simulink model "model_8264"  (R2022b)
settings: Solver=FixedStepAuto  StartTime=0.0  StopTime=2.4  FixedStep=2e-5  RelTol=1e-3
undefined symbols (not defined in the file): Acid, Lead, sigbuilder_block
libraries: spsMeanLib x24, spsVoltageMeasurementLib x18, spsGroundLib x15, spsCurrentMeasurementLib x15, spsIdealSwitchLib x12, spsSeriesRLCLoadLib x12, spsSeriesRLCBranchLib x5, spsThreePhaseVIMeasurementLib x4, simulink x4, spsPower3phInstantaneousLib x3, spsThreePhaseBreakerLib x2, slpidlib x2
(part 2 of 2)

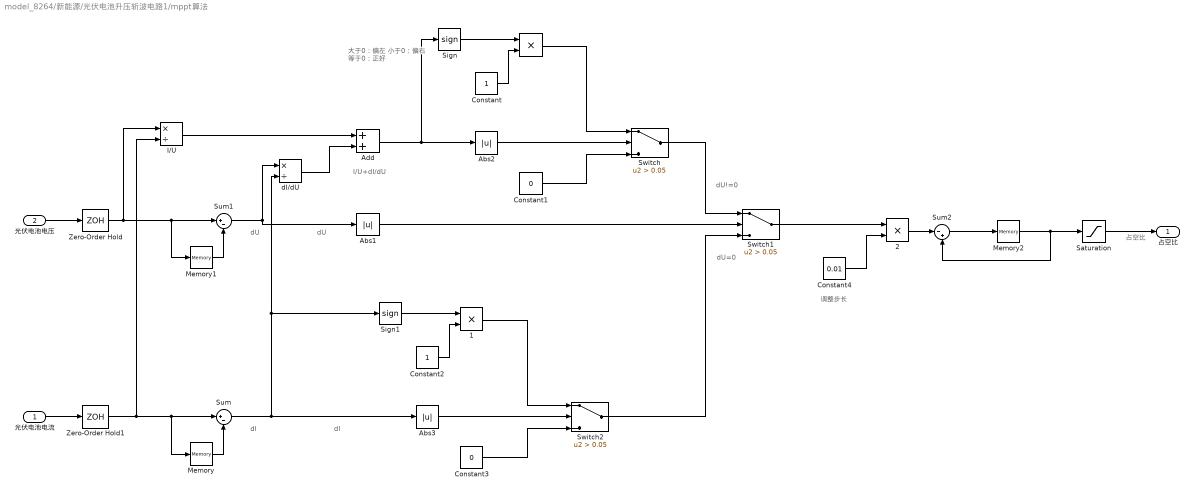
== system model_8264/新能源/光伏电池升压斩波电路1/mppt算法 ==
  note: dU!=0
  note: 占空比
  note: 调整步长
  note: 大于0：偏左
      | 小于0：偏右
      | 等于0：正好
  note: I/U+dI/dU
  note: dI
  note: dU
  note: dU
  note: dI
  note: dU=0
  光伏电池电流 : Inport
  光伏电池电压 : Inport  Port=2
  " " : Product  Inputs=**
  " 1" : Product  Inputs=**
  " 2" : Product  Inputs=**
  Abs1 : Abs  SaturateOnIntegerOverflow=off
  Abs2 : Abs  SaturateOnIntegerOverflow=off
  Abs3 : Abs  SaturateOnIntegerOverflow=off
  Add : Sum
  Constant : Constant
  Constant1 : Constant  Value=0
  Constant2 : Constant
  Constant3 : Constant  Value=0
  Constant4 : Constant  Value=0.01
  I/U : Product  Inputs=*/
  Memory : Memory
  Memory1 : Memory
  Memory2 : Memory  InitialCondition=0.5  InheritSampleTime=on
  Saturation : Saturate  UpperLimit=1  LowerLimit=0
  Sign : Signum
  Sign1 : Signum
  Sum : Sum  Inputs=|+-
  Sum1 : Sum  Inputs=|+-
  Sum2 : Sum  Inputs=|-+
  Switch : Switch  Criteria=u2 > Threshold  Threshold=0.05  SaturateOnIntegerOverflow=off  InputSameDT=off
  Switch1 : Switch  Criteria=u2 > Threshold  Threshold=0.05  SaturateOnIntegerOverflow=off  InputSameDT=off
  Switch2 : Switch  Criteria=u2 > Threshold  Threshold=0.05  SaturateOnIntegerOverflow=off  InputSameDT=off
  Zero-Order Hold : ZeroOrderHold  SampleTime=0.05
  Zero-Order Hold1 : ZeroOrderHold  SampleTime=0.05
  dI/dU : Product  Inputs=*/
  占空比 : Outport
  wires:
  光伏电池电流/1 -> Zero-Order Hold1/1
  光伏电池电压/1 -> Zero-Order Hold/1
  Zero-Order Hold1/1 -> I/U/2, Memory/1, Sum/1
  Memory/1 -> Sum/2
  Memory1/1 -> Sum1/2
  Sum1/1 -> dI/dU/1, Abs1/1
  Zero-Order Hold/1 -> I/U/1, Memory1/1, Sum1/1
  I/U/1 -> Add/1
  dI/dU/1 -> Add/2
  Add/1 -> Sign/1, Abs2/1
  Sign/1 -> " "/1
  Constant/1 -> " "/2
  Abs2/1 -> Switch/2
  Constant1/1 -> Switch/3
  " "/1 -> Switch/1
  Abs1/1 -> Switch1/2
  Switch/1 -> Switch1/1
  Sum/1 -> Abs3/1, Sign1/1, dI/dU/2
  Constant3/1 -> Switch2/3
  Constant2/1 -> " 1"/2
  Abs3/1 -> Switch2/2
  " 1"/1 -> Switch2/1
  Sign1/1 -> " 1"/1
  Switch2/1 -> Switch1/3
  Switch1/1 -> " 2"/1
  Constant4/1 -> " 2"/2
  " 2"/1 -> Sum2/1
  Sum2/1 -> Memory2/1
  Memory2/1 -> Sum2/2, Saturation/1
  Saturation/1 -> 占空比/1

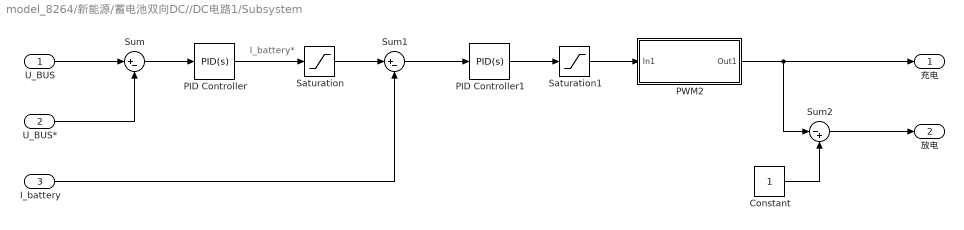
== system model_8264/新能源/蓄电池双向DC//DC电路1/Subsystem ==
  note: I_battery*
  U_BUS : Inport
  U_BUS* : Inport  Port=2
  I_battery : Inport  Port=3
  Constant : Constant
  PID Controller : slpidlib/PID Controller  Controller=PID  Form=Parallel  TimeDomain=Continuous-time  UseExternalTs=off  SampleTime=-1  IntegratorMethod=Forward Euler  FilterMethod=Forward Euler  ControllerParametersSource=internal  P=0.1  I=1  UseKiTs=off  D=0  N=100  UseFilter=on  TunerSelectOption=Transfer Function Based (PID Tuner App)  InitialConditionSource=internal  InitialConditionForIntegrator=0  InitialConditionForFilter=0  DifferentiatorICPrevScaledInput=0  ExternalReset=none  TrackingMode=off  Kt=1  LimitOutput=off  SatLimitsSource=internal  UpperSaturationLimit=inf  LowerSaturationLimit=-inf  LinearizeAsGain=on  AntiWindupMode=none  Kb=1  LimitIntegrator=off  UpperIntegratorSaturationLimit=inf  LowerIntegratorSaturationLimit=-inf  POutMin=[]  POutMax=[]  IOutMin=[]  IOutMax=[]  DOutMin=[]  DOutMax=[]  NOutMin=[]  NOutMax=[]  SumOutMin=[]  SumOutMax=[]  SaturationOutMin=[]  SaturationOutMax=[]  PParamMin=[]  PParamMax=[]  IParamMin=[]  IParamMax=[]  DParamMin=[]  DParamMax=[]  NParamMin=[]  NParamMax=[]  KbParamMin=[]  KbParamMax=[]  KtParamMin=[]  KtParamMax=[]  KbOutMin=[]  KbOutMax=[]  KtOutMin=[]  KtOutMax=[]  IntegratorOutMin=[]  IntegratorOutMax=[]  FilterOutMin=[]  FilterOutMax=[]  SumI1OutMin=[]  SumI1OutMax=[]  SumI2OutMin=[]  SumI2OutMax=[]  SumI3OutMin=[]  SumI3OutMax=[]  SumI4OutMin=[]  SumI4OutMax=[]  SumDOutMin=[]  SumDOutMax=[]  DifferentiatorOutMin=[]  DifferentiatorOutMax=[]  FilterDiffOutCoefMin=[]  FilterDiffOutCoefMax=[]  ReciprocalOutMin=[]  ReciprocalOutMax=[]  SumDenOutMin=[]  SumDenOutMax=[]  SumNumOutMin=[]  SumNumOutMax=[]  DivideOutMin=[]  DivideOutMax=[]  UdiffTsProdOutMin=[]  UdiffTsProdOutMax=[]  NTsProdOutMin=[]  NTsProdOutMax=[]  UintegralTsProdOutMin=[]  UintegralTsProdOutMax=[]  UngainTsProdOutMin=[]  UngainTsProdOutMax=[]  ClampingZeroOutDataTypeStr=Inherit: Inherit via back propagation  ClampingZeroOutMin=[]  ClampingZeroOutMax=[]  FilterDenConstantOutDataTypeStr=Inherit: Inherit via back propagation  FilterDenConstantOutMin=[]  FilterDenConstantOutMax=[]  PCopyOutDataTypeStr=Inherit: Inherit via back propagation  PCopyOutMin=[]  PCopyOutMax=[]  NCopyOutDataTypeStr=Inherit: Inherit via back propagation  NCopyOutMin=[]  NCopyOutMax=[]  IntegratorContinuousStateAttributes=''  IntegratorStateMustResolveToSignalObject=off  IntegratorRTWStateStorageClass=Auto  FilterContinuousStateAttributes=''  FilterStateMustResolveToSignalObject=off  FilterRTWStateStorageClass=Auto  ParallelPVariant=InternalParameters  IdealPVariant=Disabled  IVariant=InternalParameters  DVariant=InternalParameters  IntegratorVariant=Continuous  SatVariant=Disabled  AWVariant=Passthrough  PCopyVariant=Disabled  TRVariant=Disabled  FdbkBlocksVariant=Forward  IdealPFdbkVariant=Disabled  SatFdbkVariant=Disabled  DerivativeFilterVariant=ContFilter  NVariant=InternalParameters  NCopyVariant=Disabled  FilterICVariant=InternalICsFilter  IntegratorICVariant=InternalICs  ExternalResetVariant=Disabled  TRSumVariant=Passthrough  SumFdbkVariant=Disabled  SumVariant=Sum_PID  TsampFilterVariant=InternalTs  TsampNgainVariant=Passthrough  TsampIntegralVariant=Passthrough  ExternalSaturationOutDataTypeStr=Inherit: Same as second input
  PID Controller1 : slpidlib/PID Controller  Controller=PID  Form=Parallel  TimeDomain=Continuous-time  UseExternalTs=off  SampleTime=-1  IntegratorMethod=Forward Euler  FilterMethod=Forward Euler  ControllerParametersSource=internal  P=0.02  I=1  UseKiTs=off  D=0  N=100  UseFilter=on  TunerSelectOption=Transfer Function Based (PID Tuner App)  InitialConditionSource=internal  InitialConditionForIntegrator=0  InitialConditionForFilter=0  DifferentiatorICPrevScaledInput=0  ExternalReset=none  TrackingMode=off  Kt=1  LimitOutput=off  SatLimitsSource=internal  UpperSaturationLimit=inf  LowerSaturationLimit=-inf  LinearizeAsGain=on  AntiWindupMode=none  Kb=1  LimitIntegrator=off  UpperIntegratorSaturationLimit=inf  LowerIntegratorSaturationLimit=-inf  POutMin=[]  POutMax=[]  IOutMin=[]  IOutMax=[]  DOutMin=[]  DOutMax=[]  NOutMin=[]  NOutMax=[]  SumOutMin=[]  SumOutMax=[]  SaturationOutMin=[]  SaturationOutMax=[]  PParamMin=[]  PParamMax=[]  IParamMin=[]  IParamMax=[]  DParamMin=[]  DParamMax=[]  NParamMin=[]  NParamMax=[]  KbParamMin=[]  KbParamMax=[]  KtParamMin=[]  KtParamMax=[]  KbOutMin=[]  KbOutMax=[]  KtOutMin=[]  KtOutMax=[]  IntegratorOutMin=[]  IntegratorOutMax=[]  FilterOutMin=[]  FilterOutMax=[]  SumI1OutMin=[]  SumI1OutMax=[]  SumI2OutMin=[]  SumI2OutMax=[]  SumI3OutMin=[]  SumI3OutMax=[]  SumI4OutMin=[]  SumI4OutMax=[]  SumDOutMin=[]  SumDOutMax=[]  DifferentiatorOutMin=[]  DifferentiatorOutMax=[]  FilterDiffOutCoefMin=[]  FilterDiffOutCoefMax=[]  ReciprocalOutMin=[]  ReciprocalOutMax=[]  SumDenOutMin=[]  SumDenOutMax=[]  SumNumOutMin=[]  SumNumOutMax=[]  DivideOutMin=[]  DivideOutMax=[]  UdiffTsProdOutMin=[]  UdiffTsProdOutMax=[]  NTsProdOutMin=[]  NTsProdOutMax=[]  UintegralTsProdOutMin=[]  UintegralTsProdOutMax=[]  UngainTsProdOutMin=[]  UngainTsProdOutMax=[]  ClampingZeroOutDataTypeStr=Inherit: Inherit via back propagation  ClampingZeroOutMin=[]  ClampingZeroOutMax=[]  FilterDenConstantOutDataTypeStr=Inherit: Inherit via back propagation  FilterDenConstantOutMin=[]  FilterDenConstantOutMax=[]  PCopyOutDataTypeStr=Inherit: Inherit via back propagation  PCopyOutMin=[]  PCopyOutMax=[]  NCopyOutDataTypeStr=Inherit: Inherit via back propagation  NCopyOutMin=[]  NCopyOutMax=[]  IntegratorContinuousStateAttributes=''  IntegratorStateMustResolveToSignalObject=off  IntegratorRTWStateStorageClass=Auto  FilterContinuousStateAttributes=''  FilterStateMustResolveToSignalObject=off  FilterRTWStateStorageClass=Auto  ParallelPVariant=InternalParameters  IdealPVariant=Disabled  IVariant=InternalParameters  DVariant=InternalParameters  IntegratorVariant=Continuous  SatVariant=Disabled  AWVariant=Passthrough  PCopyVariant=Disabled  TRVariant=Disabled  FdbkBlocksVariant=Forward  IdealPFdbkVariant=Disabled  SatFdbkVariant=Disabled  DerivativeFilterVariant=ContFilter  NVariant=InternalParameters  NCopyVariant=Disabled  FilterICVariant=InternalICsFilter  IntegratorICVariant=InternalICs  ExternalResetVariant=Disabled  TRSumVariant=Passthrough  SumFdbkVariant=Disabled  SumVariant=Sum_PID  TsampFilterVariant=InternalTs  TsampNgainVariant=Passthrough  TsampIntegralVariant=Passthrough  ExternalSaturationOutDataTypeStr=Inherit: Same as second input
  PWM2 : Subsystem
  Saturation : Saturate  UpperLimit=40  LowerLimit=-40
  Saturation1 : Saturate  UpperLimit=0.95  LowerLimit=0.05
  Sum : Sum  Inputs=|+-
  Sum1 : Sum  Inputs=|+-
  Sum2 : Sum  Inputs=|-+
  充电 : Outport
  放电 : Outport  Port=2
  wires:
  U_BUS/1 -> Sum/1
  U_BUS*/1 -> Sum/2
  PID Controller/1 -> Saturation/1
  Sum/1 -> PID Controller/1
  Saturation/1 -> Sum1/1
  I_battery/1 -> Sum1/2
  Sum1/1 -> PID Controller1/1
  PID Controller1/1 -> Saturation1/1
  Constant/1 -> Sum2/2
  PWM2/1(Out1) -> Sum2/1, 充电/1
  Sum2/1 -> 放电/1
  Saturation1/1 -> PWM2/1(In1)

== system model_8264/新能源/蓄电池双向DC//DC电路1/Subsystem/PWM2 ==
  In1 : Inport
  Constant : Constant
  Constant1 : Constant  Value=0
  Repeating Sequence : simulink/Sources/Repeating Sequence  rep_seq_t=[0 1e-4]  rep_seq_y=[0 2]
  Saturation : Saturate  UpperLimit=1  LowerLimit=0
  Scope : Scope  NumInputPorts=2
  Sum : Sum  Inputs=|+-
  Switch : Switch  Criteria=u2 > Threshold  SaturateOnIntegerOverflow=off  InputSameDT=off
  Zero-Order Hold : ZeroOrderHold  SampleTime=0.05
  Out1 : Outport
  wires:
  In1/1 -> Zero-Order Hold/1
  Zero-Order Hold/1 -> Saturation/1
  Switch/1 -> Scope/1, Out1/1
  Constant/1 -> Switch/1
  Constant1/1 -> Switch/3
  Saturation/1 -> Sum/1
  Sum/1 -> Switch/2
  Repeating Sequence/1 -> Scope/2, Sum/2

== matlab function model_8264/新负荷3/电灯的使用曲线 input:当前时间点 output:开启状态 ==
  data: u input; y output
function y = fcn(u)
    if u>0.6&&u<2.1
        y=1;
    else
        y=0;
    end
end

== matlab function model_8264/新负荷3/电饭锅的使用曲线 input:当前时间点 output:开启状态 ==
  data: u input; y output
function y = fcn(u)
    if u>1.9&&u<2.1
        y=1;
    else
        y=0;
    end
end

== matlab function model_8264/新负荷3/空调的使用曲线 input:当前时间点 output:开启状态 ==
  data: u input; y output
function y = fcn(u)
    if u>1.5&&u<2.1
        y=1;
    else
        y=0;
    end
end

== matlab function model_8264/新负荷3/洗衣机的使用曲线 input:当前时间点 output:开启状态1 ==
  data: u input; y output
function y = fcn(u)
    if u>1.0&&u<2.1
        y=1;
    else
        y=0;
    end
end

== matlab function model_8264/新负荷3/电灯的使用曲线 input:当前时间点 output:开启状态1 ==
  data: u input; y output
function y = fcn(u)
    if u>0.6&&u<2.1
        y=1;
    else
        y=0;
    end
end

== matlab function model_8264/新负荷3/电饭锅的使用曲线 input:当前时间点 output:开启状态1 ==
  data: u input; y output
function y = fcn(u)
    if u>1.9&&u<2.1
        y=1;
    else
        y=0;
    end
end

== matlab function model_8264/新负荷3/空调的使用曲线 input:当前时间点 output:开启状态1 ==
  data: u input; y output
function y = fcn(u)
    if u>1.5&&u<2.1
        y=1;
    else
        y=0;
    end
end

== matlab function model_8264/新负荷3/洗衣机的使用曲线 input:当前时间点 output:开启状态2 ==
  data: u input; y output
function y = fcn(u)
    if u>1.0&&u<2.1
        y=1;
    else
        y=0;
    end
end

== matlab function model_8264/新负荷3/洗衣机的使用曲线 input:当前时间点 output:开启状态 ==
  data: u input; y output
function y = fcn(u)
    if u>1.0&&u<2.1
        y=1;
    else
        y=0;
    end
end

== matlab function model_8264/新负荷3/电灯的使用曲线 input:当前时间点 output:开启状态2 ==
  data: u input; y output
function y = fcn(u)
    if u>0.6&&u<2.1
        y=1;
    else
        y=0;
    end
end

== matlab function model_8264/新负荷3/电饭锅的使用曲线 input:当前时间点 output:开启状态2 ==
  data: u input; y output
function y = fcn(u)
    if u>1.9&&u<2.1
        y=1;
    else
        y=0;
    end
end

== matlab function model_8264/新负荷3/空调的使用曲线 input:当前时间点 output:开启状态2 ==
  data: u input; y output
function y = fcn(u)
    if u>1.5&&u<2.1
        y=1;
    else
        y=0;
    end
end
